simulink model "verify_Kinematic_Viscosity2_mdl"  (R2013b)
settings: Solver=ode45  SolverMode=SingleTasking  StartTime=0.0  StopTime=10.0  RelTol=1e-3
libraries: carnot x2, simulink x1
settings Model: CovMetricSettings=dwe  CovHtmlReporting=off  covSaveCumulativeToWorkspaceVar=off  CovSaveSingleToWorkspaceVar=off  CovExternalEMLEnable=on  Creator=darl  LastModifiedBy=drhf
settings DataIOCC: LimitDataPoints=off
settings DebuggingCC: UnderspecifiedInitializationDetection=Simplified  MergeDetectMultiDrivingBlocksExec=error  SolverPrmCheckMsg=none  FrameProcessingCompatibilityMsg=error  SFUnexpectedBacktrackingDiag=error  SFNoUnconditionalDefaultTransitionDiag=error
settings HardwareCC: ProdBitPerPointer=64  ProdLargestAtomicFloat=Float  ProdIntDivRoundTo=Zero  ProdEndianess=LittleEndian  ProdHWDeviceType=Specified
settings ModelReferenceCC: PropagateSignalLabelsOutOfModel=on
settings GRTTargetCC: CodeReplacementLibrary=C99 (ISO)  GeneratePreprocessorConditionals=Use local settings

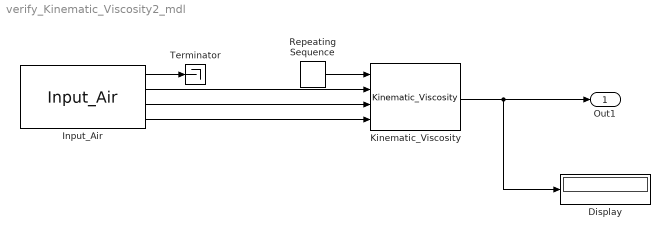
== system verify_Kinematic_Viscosity2_mdl ==
  Display : Display
  Input_Air : carnot/Basic/Material_Properties/Input_Air  T=20  p=1e5  x=0
  Kinematic_Viscosity : carnot/Basic/Material_Properties/Kinematic_Viscosity  VariantControl=CarlibClassic  INPUTARGUMENTS=state variables (classic)  DEBUGLEVEL=WARNINGLEVEL  MAXTOTALMESSAGES=inf  MAXCONSECUTIVEMESSAGES=inf  WRITETOFILE=0  FILENAME='errors.txt'
  Repeating Sequence : simulink/Sources/Repeating Sequence  rep_seq_t=0:6  rep_seq_y=[2 27 52 77 102 127 152]
  Terminator : Terminator
  Out1 : Outport
  wires:
  Input_Air/4 -> Kinematic_Viscosity/4
  Input_Air/2 -> Kinematic_Viscosity/2
  Input_Air/3 -> Kinematic_Viscosity/3
  Input_Air/1 -> Terminator/1
  Repeating Sequence/1 -> Kinematic_Viscosity/1
  Kinematic_Viscosity/1 -> Out1/1, Display/1
